simulink model "Resetable_Subsystem"  (R2017b)
settings: Solver=FixedStepDiscrete  StartTime=0.0  StopTime=10.0  FixedStep=0.200000  RelTol=1e-3
settings Model: Creator=hbourbou  LastModifiedBy=hbourbou
settings DataIOCC: SaveFormat=StructureWithTime
settings OptimizationCC: LifeSpan=inf
settings DebuggingCC: SFExecutionAtInitializationDiag=none
settings HardwareCC: ProdBitPerSizeT=32  ProdBitPerPtrDiffT=32  ProdWordSize=32  ProdHWDeviceType=Specified
settings CodeAppCC: StateflowObjectComments=on

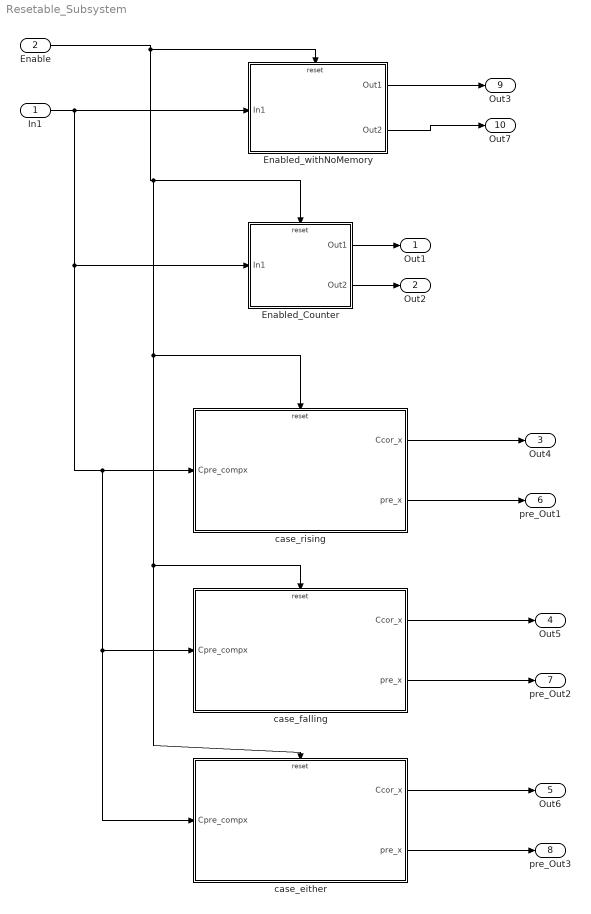
== system Resetable_Subsystem ==
  In1 : Inport
  Enable : Inport  Port=2
  Enabled_Counter : Subsystem  TreatAsAtomicUnit=on
  Enabled_withNoMemory : Subsystem  TreatAsAtomicUnit=on
  case_either : Subsystem  TreatAsAtomicUnit=on
  case_falling : Subsystem  TreatAsAtomicUnit=on
  case_rising : Subsystem  TreatAsAtomicUnit=on
  Out1 : Outport
  Out2 : Outport  Port=2
  Out4 : Outport  Port=3
  Out5 : Outport  Port=4
  Out6 : Outport  Port=5
  pre_Out1 : Outport  Port=6
  pre_Out2 : Outport  Port=7
  pre_Out3 : Outport  Port=8
  Out3 : Outport  Port=9
  Out7 : Outport  Port=10
  wires:
  Enabled_Counter/1(Out1) -> Out1/1
  Enabled_Counter/2(Out2) -> Out2/1
  Enable/1 -> Enabled_Counter/Reset, case_rising/Reset, case_falling/Reset, case_either/Reset, Enabled_withNoMemory/Reset
  case_rising/1(Ccor_x) -> Out4/1
  In1/1 -> Enabled_withNoMemory/1(In1), Enabled_Counter/1(In1), case_either/1(Cpre_compx), case_falling/1(Cpre_compx), case_rising/1(Cpre_compx)
  case_falling/1(Ccor_x) -> Out5/1
  case_either/1(Ccor_x) -> Out6/1
  case_rising/2(pre_x) -> pre_Out1/1
  case_falling/2(pre_x) -> pre_Out2/1
  case_either/2(pre_x) -> pre_Out3/1
  Enabled_withNoMemory/1(Out1) -> Out3/1
  Enabled_withNoMemory/2(Out2) -> Out7/1

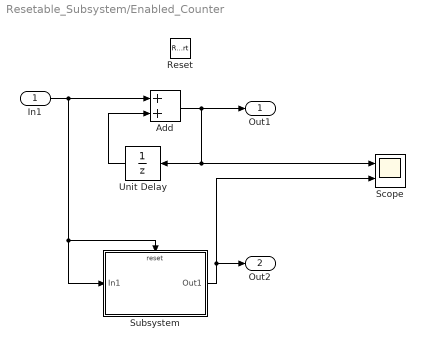
== system Resetable_Subsystem/Enabled_Counter ==
  In1 : Inport
  Reset : ResetPort  DisableCoverage=on
  Add : Sum
  Scope : Scope  NumInputPorts=2
  Subsystem : Subsystem  TreatAsAtomicUnit=on
  Unit Delay : UnitDelay  SampleTime=-1
  Out1 : Outport  OutputWhenDisabled=reset  InitialOutput=0
  Out2 : Outport  Port=2
  wires:
  Unit Delay/1 -> Add/2
  Subsystem/1(Out1) -> Scope/2, Out2/1
  In1/1 -> Subsystem/Reset, Subsystem/1(In1), Add/1
  Add/1 -> Scope/1, Unit Delay/1, Out1/1

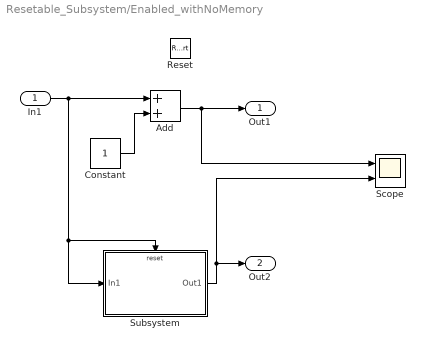
== system Resetable_Subsystem/Enabled_withNoMemory ==
  In1 : Inport
  Reset : ResetPort  DisableCoverage=on
  Add : Sum
  Constant : Constant
  Scope : Scope  NumInputPorts=2
  Subsystem : Subsystem  TreatAsAtomicUnit=on
  Out1 : Outport  OutputWhenDisabled=reset  InitialOutput=0
  Out2 : Outport  Port=2
  wires:
  Subsystem/1(Out1) -> Scope/2, Out2/1
  In1/1 -> Subsystem/Reset, Subsystem/1(In1), Add/1
  Add/1 -> Scope/1, Out1/1
  Constant/1 -> Add/2

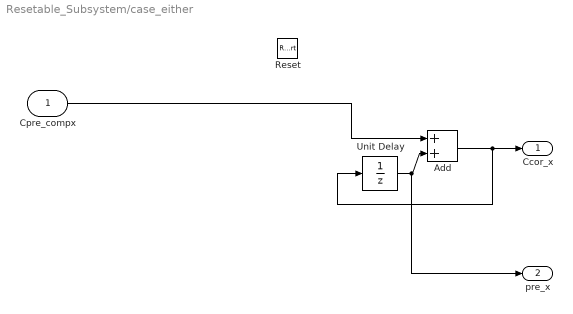
== system Resetable_Subsystem/case_either ==
  Cpre_compx : Inport  OutDataTypeStr=double  PortDimensions=[1]
  Reset : ResetPort  DisableCoverage=on  ResetTriggerType=either
  Add : Sum
  Unit Delay : UnitDelay  SampleTime=-1.0000000000000000
  Ccor_x : Outport  InitialOutput=0
  pre_x : Outport  Port=2  InitialOutput=0
  wires:
  Cpre_compx/1 -> Add/1
  Add/1 -> Unit Delay/1, Ccor_x/1
  Unit Delay/1 -> pre_x/1, Add/2

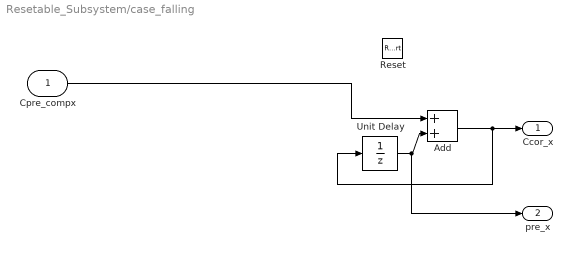
== system Resetable_Subsystem/case_falling ==
  Cpre_compx : Inport  OutDataTypeStr=double  PortDimensions=[1]
  Reset : ResetPort  DisableCoverage=on  ResetTriggerType=falling
  Add : Sum
  Unit Delay : UnitDelay  SampleTime=-1.0000000000000000
  Ccor_x : Outport  OutputWhenDisabled=reset  InitialOutput=0
  pre_x : Outport  Port=2  InitialOutput=0
  wires:
  Cpre_compx/1 -> Add/1
  Add/1 -> Unit Delay/1, Ccor_x/1
  Unit Delay/1 -> pre_x/1, Add/2

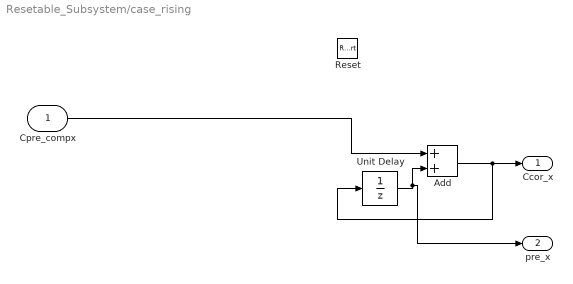
== system Resetable_Subsystem/case_rising ==
  Cpre_compx : Inport  OutDataTypeStr=double  PortDimensions=[1]
  Reset : ResetPort  DisableCoverage=on
  Add : Sum
  Unit Delay : UnitDelay  SampleTime=-1.0000000000000000
  Ccor_x : Outport  InitialOutput=0
  pre_x : Outport  Port=2  InitialOutput=0
  wires:
  Cpre_compx/1 -> Add/1
  Unit Delay/1 -> pre_x/1, Add/2
  Add/1 -> Unit Delay/1, Ccor_x/1

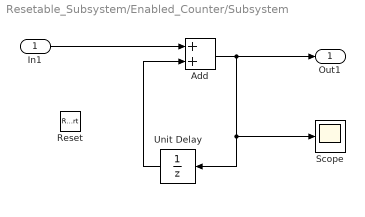
== system Resetable_Subsystem/Enabled_Counter/Subsystem ==
  In1 : Inport
  Reset : ResetPort  DisableCoverage=on
  Add : Sum
  Scope : Scope
  Unit Delay : UnitDelay  SampleTime=-1
  Out1 : Outport
  wires:
  In1/1 -> Add/1
  Unit Delay/1 -> Add/2
  Add/1 -> Scope/1, Unit Delay/1, Out1/1

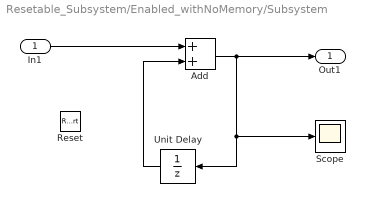
== system Resetable_Subsystem/Enabled_withNoMemory/Subsystem ==
  In1 : Inport
  Reset : ResetPort  DisableCoverage=on
  Add : Sum
  Scope : Scope
  Unit Delay : UnitDelay  SampleTime=-1
  Out1 : Outport
  wires:
  In1/1 -> Add/1
  Unit Delay/1 -> Add/2
  Add/1 -> Scope/1, Unit Delay/1, Out1/1
